simulink model "ex_bus_tutorial_virtual"  (R2017b)
settings: Solver=FixedStepDiscrete  StartTime=0.0  StopTime=10.0  FixedStep=0.200000  RelTol=1e-3
PreLoadFcn:
  | % Bus object: subBus
  | clear elems;
  | elems(1) = Simulink.BusElement;
  | elems(1).Name = 'chirp';
  | elems(1).Dimensions = 2;
  | elems(1).DimensionsMode = 'Fixed';
  | elems(1).DataType = 'double';
  | elems(1).SampleTime = -1;
  | elems(1).Complexity = 'real';
  | elems(1).Min = [];
  | elems(1).Max = [];
  | elems(1).DocUnits = '';
  | elems(1).Description = '';
  | 
  | elems(2) = Simulink.BusElement;
  | elems(2).Name = 'sine';
  | elems(2).Dimensions = 3;
  | elems(2).DimensionsMode = 'Fixed';
  | elems(2).DataType = 'int32';
  | elems(2).SampleTime = -1;
  | elems(2).Complexity = 'real';
  | elems(2).Min = [];
  | elems(2).Max = [];
  | elems(2).DocUnits = '';
  | elems(2).Description = '';
  | 
  | subBus = Simulink.Bus;
  | subBus.HeaderFile = '';
  | subBus.Description = '';
  | subBus.DataScope = 'Auto';
  | subBus.Alignment = -1;
  | subBus.Elements = elems;
  | clear elems;
  | assignin('base','subBus', subBus);
  | 
  | % Bus object: topBus
  | clear elems;
  | elems(1) = Simulink.BusElement;
  | elems(1).Name = 'subSignal';
  | elems(1).Dimensions = 1;
  | elems(1).DimensionsMode = 'Fixed';
  | elems(1).DataType = 'Bus: subBus';
  | elems(1).SampleTime = -1;
  | elems(1).Complexity = 'real';
  | elems(1).Min = [];
  | elems(1).Max = [];
  | elems(1).DocUnits = '';
  | elems(1).Description = '';
  | 
  | elems(2) = Simulink.BusElement;
  | elems(2).Name = 'step';
  | elems(2).Dimensions = 4;
  | elems(2).DimensionsMode = 'Fixed';
  | elems(2).DataType = 'boolean';
  | elems(2).SampleTime = -1;
  | elems(2).Complexity = 'real';
  | elems(2).Min = [];
  | elems(2).Max = [];
  | elems(2).DocUnits = '';
  | elems(2).Description = '';
  | 
  | topBus = Simulink.Bus;
  | topBus.HeaderFile = '';
  | topBus.Description = '';
  | topBus.DataScope = 'Auto';
  | topBus.Alignment = -1;
  | topBus.Elements = elems;
  | clear elems;
  | assignin('base','topBus', topBus);
settings Model: Creator=The MathWorks, Inc.  LastModifiedBy=hbourbou
settings OptimizationCC: LifeSpan=inf
settings DebuggingCC: SFExecutionAtInitializationDiag=none
settings HardwareCC: ProdBitPerSizeT=32  ProdBitPerPtrDiffT=32  ProdWordSize=32  ProdHWDeviceType=Specified
settings CodeAppCC: StateflowObjectComments=on
settings ConfigComp: CovMetricSettings=dswe

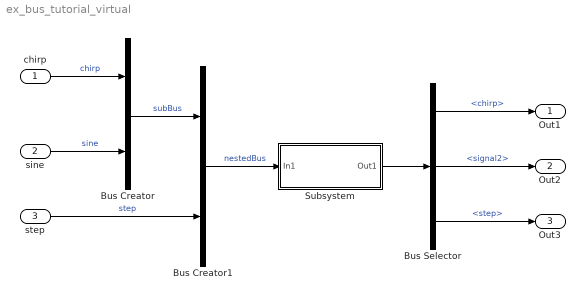
== system ex_bus_tutorial_virtual ==
  chirp : Inport  OutDataTypeStr=double
  sine : Inport  Port=2  OutDataTypeStr=int32
  step : Inport  Port=3  OutDataTypeStr=boolean  PortDimensions=4
  Bus Creator1 : BusCreator  Inputs=2
      settings: AttributesFormatString=NestedBus
  Bus Selector : BusSelector  OutputSignals=signal1.chirp,signal1.signal2,step
      settings: AttributesFormatString=Bus Selector
  Bus Creator : BusCreator  Inputs=2
      settings: AttributesFormatString=SubBus
  Subsystem : Subsystem
  Out1 : Outport
  Out2 : Outport  Port=2
  Out3 : Outport  Port=3
  wires:
  chirp/1 -> Bus Creator/1  "chirp"
  Bus Creator/1 -> Bus Creator1/1  "subBus"
  Bus Creator1/1 -> Subsystem/1(In1)  "nestedBus"
  sine/1 -> Bus Creator/2  "sine"
  step/1 -> Bus Creator1/2  "step"
  Subsystem/1(Out1) -> Bus Selector/1
  Bus Selector/1 -> Out1/1  "<chirp>"
  Bus Selector/2 -> Out2/1  "<signal2>"
  Bus Selector/3 -> Out3/1  "<step>"

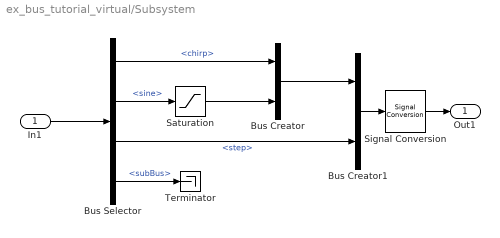
== system ex_bus_tutorial_virtual/Subsystem ==
  In1 : Inport
  Bus Selector : BusSelector  OutputSignals=subBus.chirp,subBus.sine,step,subBus
      settings: AttributesFormatString=Bus Selector
  Bus Creator : BusCreator  Inputs=2
  Bus Creator1 : BusCreator  Inputs=2
  Saturation : Saturate  LowerLimit=-5
  Signal Conversion : SignalConversion  ConversionOutput=Nonvirtual bus  OutDataTypeStr=Bus: topBus  OverrideOpt=off
  Terminator : Terminator
  Out1 : Outport
  wires:
  In1/1 -> Bus Selector/1
  Bus Selector/1 -> Bus Creator/1  "<chirp>"
  Bus Selector/2 -> Saturation/1  "<sine>"
  Saturation/1 -> Bus Creator/2
  Bus Selector/3 -> Bus Creator1/2  "<step>"
  Bus Creator/1 -> Bus Creator1/1
  Bus Creator1/1 -> Signal Conversion/1
  Signal Conversion/1 -> Out1/1
  Bus Selector/4 -> Terminator/1  "<subBus>"
